simulink model "Task2_sim"  (R2014a)
settings: Solver=ode45  StartTime=0.0  StopTime=1  RelTol=1e-3
settings Model: Creator=bunka  LastModifiedBy=bunka

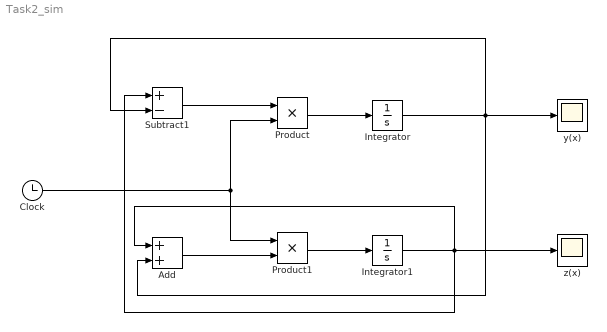
== system Task2_sim ==
  Add : Sum
  Clock : Clock
  Integrator : Integrator  InitialCondition=1
  Integrator1 : Integrator  InitialCondition=1
  Product : Product
  Product1 : Product
  Subtract1 : Sum  Inputs=+-
  y(x) : Scope
  z(x) : Scope
  wires:
  Integrator1/1 -> Subtract1/1, Add/1, z(x)/1
  Integrator/1 -> Add/2, Subtract1/2, y(x)/1
  Product/1 -> Integrator/1
  Product1/1 -> Integrator1/1
  Subtract1/1 -> Product/1
  Add/1 -> Product1/2
  Clock/1 -> Product/2, Product1/1
